simulink model "RI_DIERR"  (R2013b)
settings: Solver=ode45  StartTime=0.0  StopTime=10.0  MaxStep=1e-3  RelTol=1e-3
InitFcn:
  | K = 1;
  | tau = 1;
  | 
  | T_S = 50e-3;
libraries: simulink x1
settings Model: Creator=Szalay  LastModifiedBy=Szalay

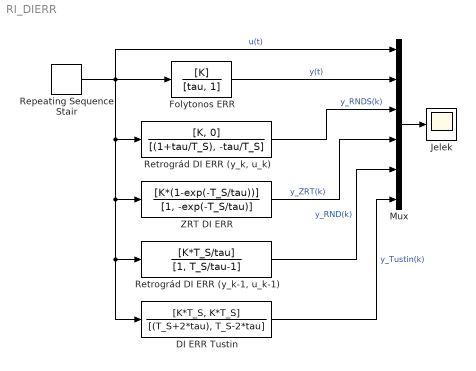
== system RI_DIERR ==
  DI ERR Tustin : DiscreteTransferFcn  Numerator=[K*T_S, K*T_S]  Denominator=[(T_S+2*tau), T_S-2*tau]  SampleTime=T_S
  Folytonos ERR : TransferFcn  Numerator=[K]  Denominator=[tau, 1]
  Jelek : Scope
      settings: ShowLegends=on
  Mux : Mux  Inputs=6
  Repeating Sequence Stair : simulink/Sources/Repeating Sequence Stair  OutValues=[1, 3, -4, 2, -1]  tsamp=2  OutMin=[]  OutMax=[]  OutDataTypeStr=double  OutputDataTypeScalingMode=double  OutDataType=fixdt(0,8)  ConRadixGroup=Best Precision: Vector-wise  OutScaling=2^-12
  "Retrográd DI ERR (y_k, u_k)" : DiscreteTransferFcn  Numerator=[K, 0]  Denominator=[(1+tau/T_S), -tau/T_S]  SampleTime=T_S
  "Retrográd DI ERR (y_k-1, u_k-1)" : DiscreteTransferFcn  Numerator=[K*T_S/tau]  Denominator=[1, T_S/tau-1]  SampleTime=T_S
  ZRT DI ERR : DiscreteTransferFcn  Numerator=[K*(1-exp(-T_S/tau))]  Denominator=[1, -exp(-T_S/tau)]  SampleTime=T_S
  wires:
  Repeating Sequence Stair/1 -> Folytonos ERR/1, Mux/1, DI ERR Tustin/1, "Retrográd DI ERR (y_k-1, u_k-1)"/1, ZRT DI ERR/1, "Retrográd DI ERR (y_k, u_k)"/1  "u(t)"
  Folytonos ERR/1 -> Mux/2  "y(t)"
  Mux/1 -> Jelek/1
  "Retrográd DI ERR (y_k, u_k)"/1 -> Mux/3  "y_RNDS(k)"
  ZRT DI ERR/1 -> Mux/4  "y_ZRT(k)"
  "Retrográd DI ERR (y_k-1, u_k-1)"/1 -> Mux/5  "y_RND(k)"
  DI ERR Tustin/1 -> Mux/6  "y_Tustin(k)"
